simulink model "ControlLabPracticeSS"  (R2020b)
settings: Solver=VariableStepAuto  StartTime=0.0  StopTime=10.0  RelTol=1e-3
values from neighbouring files (symbols this model uses):
  A = [0 1 0 0 0; -k/J1 -(b+Bv)/J1 k/J1 b/J1 Kt/J1; 0 0 0 1 0; k/J2 b/J2 -k/J2 -b/J2 0; 0 -Ke/La 0 0 -Ra/La]    [ControlLabPractice.m]
  B = [0; 0; 0; 0; 1/La]    [ControlLabPractice.m]
  C = [1 0 0 0 0; 0 0 1 0 0; 0 0 0 0 1]    [ControlLabPractice.m]
  D = [0; 0; 0]    [ControlLabPractice.m]
settings Model: Creator=auamai  LastModifiedBy=auamai

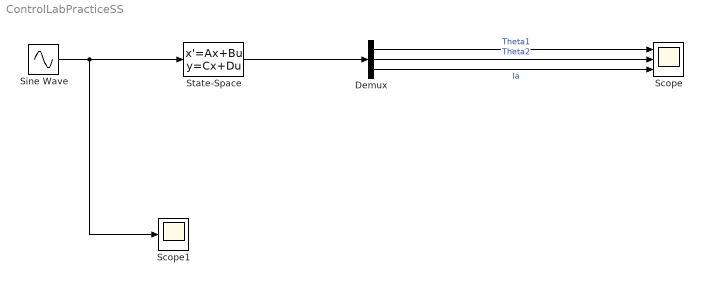
== system ControlLabPracticeSS ==
  Demux : Demux  Outputs=3
  Scope : Scope  NumInputPorts=3
  Scope1 : Scope
  Sine Wave : Sin  Frequency=20  SampleTime=0
  State-Space : StateSpace  A=A  B=B  C=C  D=D  InitialCondition=0
  wires:
  Sine Wave/1 -> Scope1/1, State-Space/1
  State-Space/1 -> Demux/1
  Demux/1 -> Scope/1  "Theta1"
  Demux/2 -> Scope/2  "Theta2"
  Demux/3 -> Scope/3  "Ia"
